simulink model "modelo_no_lineal"  (R2013b)
settings: Solver=ode45  StartTime=0.0  StopTime=10  RelTol=1e-3
values from neighbouring files (symbols this model uses):
  g = 9.8    [modelo_lineal_controlado.m]    (also in parametros_fisicos.m)
  L = 0.3    [modelo_lineal_controlado.m]    (also in parametros_fisicos.m = 0.2)
  M = 2    [modelo_lineal_controlado.m]    (also in parametros_fisicos.m)
  m = 0.1    [modelo_lineal_controlado.m]    (also in parametros_fisicos.m = 0.001)
settings Model: Creator=Julian  LastModifiedBy=Julian

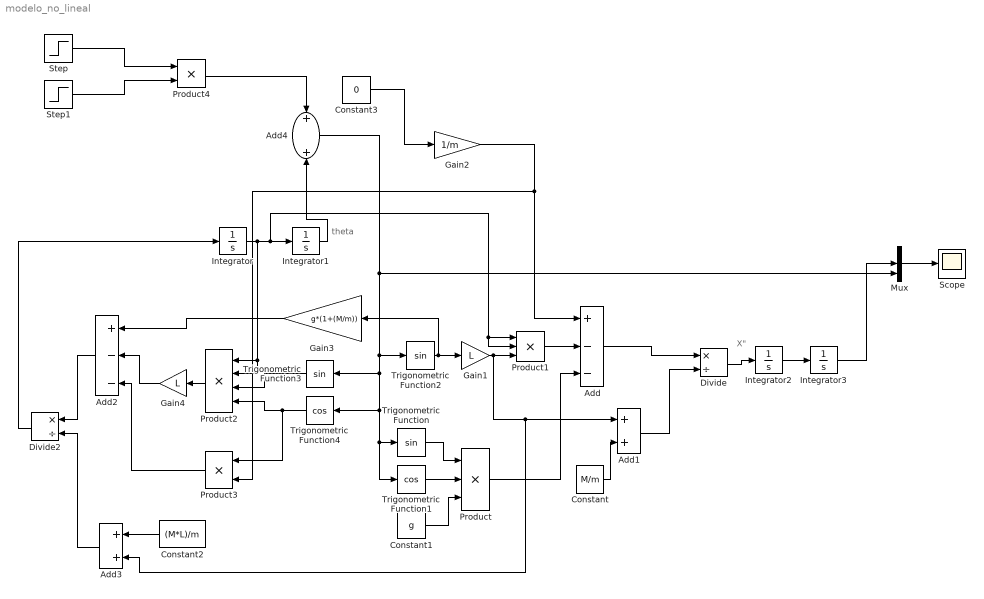
== system modelo_no_lineal ==
  note: theta
  note: X"
  Add : Sum  Inputs=+--
  Add1 : Sum
  Add2 : Sum  Inputs=+--
  Add3 : Sum
  Add4 : Sum
  Constant : Constant  Value=M/m
  Constant1 : Constant  Value=g
  Constant2 : Constant  Value=(M*L)/m
  Constant3 : Constant  Value=0
  Divide : Product  Inputs=*/
  Divide2 : Product  Inputs=*/
  Gain1 : Gain  Gain=L
  Gain2 : Gain  Gain=1/m
  Gain3 : Gain  Gain=g*(1+(M/m))
  Gain4 : Gain  Gain=L
  Integrator{,1..3} (4 alike) : Integrator
  Mux : Mux  Inputs=3
  Product : Product  Inputs=3
  Product1 : Product  Inputs=3
  Product2 : Product  Inputs=4
  Product3 : Product
  Product4 : Product
  Scope : Scope
  Step : Step  Time=2  Before=1  After=0  SampleTime=0
  Step1 : Step  SampleTime=0
  Trigonometric Function : Trigonometry
  Trigonometric Function1 : Trigonometry  Operator=cos
  Trigonometric Function2 : Trigonometry
  Trigonometric Function3 : Trigonometry
  Trigonometric Function4 : Trigonometry  Operator=cos
  wires:
  Trigonometric Function1/1 -> Product/2
  Trigonometric Function/1 -> Product/1
  Product/1 -> Add/3
  Trigonometric Function2/1 -> Gain3/1, Gain1/1
  Gain1/1 -> Add3/2, Add1/1, Product1/3
  Product1/1 -> Add/2
  Integrator/1 -> Product2/1, Product2/2, Product1/1, Product1/2, Integrator1/1
  Constant/1 -> Add1/2
  Add/1 -> Divide/1
  Add1/1 -> Divide/2
  Constant1/1 -> Product/3
  Product2/1 -> Gain4/1
  Trigonometric Function4/1 -> Product3/1, Product2/4
  Trigonometric Function3/1 -> Product2/3
  Gain2/1 -> Product3/2, Add/1
  Gain3/1 -> Add2/1
  Gain4/1 -> Add2/2
  Product3/1 -> Add2/3
  Divide/1 -> Integrator2/1
  Integrator2/1 -> Integrator3/1
  Integrator3/1 -> Mux/2
  Add2/1 -> Divide2/1
  Add3/1 -> Divide2/2
  Constant2/1 -> Add3/1
  Divide2/1 -> Integrator/1
  Step/1 -> Product4/1
  Step1/1 -> Product4/2
  Mux/1 -> Scope/1
  Constant3/1 -> Gain2/1
  Add4/1 -> Mux/3, Trigonometric Function2/1, Trigonometric Function3/1, Trigonometric Function/1, Trigonometric Function1/1, Trigonometric Function4/1
  Product4/1 -> Add4/1
  Integrator1/1 -> Add4/2
